simulink model "adcs_v16_integral_light_sun_sgp_igrf"  (Simulink 7.4)
settings: Solver=ode4  StartTime=0.0  StopTime=5000  FixedStep=s_SIM_STEP_SIZE  RelTol=1e-3
values from neighbouring files (symbols this model uses):
  A = ((T_SIDE + .29)*1e-3)^2    [constants_v13.m]    (also in constants_v15.m; constants_v15_Pow.m; constants_v15_Pow_ss_error.m; constants_v16_integral_kartavya.m)
  Bstar = SGP4dragp    (= -3.5889e-05)    [constants_v16_integral_light_sun_sgp_igrf_power_13Dec2011.m]    (also in getOrbitData.m = SGP4dragp; sgp.m = modTLE(4))
  Ca_Solar_Drag = 1.4    [constants_v13.m]    (also in constants_v15.m; constants_v15_Pow.m; constants_v15_Pow_ss_error.m; constants_v16_integral_kartavya.m)
  Cd = 2.2    [constants_v13.m]    (also in constants_v15.m; constants_v15_Pow.m; constants_v15_Pow_ss_error.m; constants_v16_integral_kartavya.m)
  check_time = 60000    [constants_v13.m]    (also in constants_v15.m = 10000; constants_v15_Pow.m = 10000; constants_v15_Pow_ss_error.m = 10000; constants_v16_integral_kartavya.m = 10000)
  ddn0 = 6*2*pi*SGPdragp2/(1440^3)    (= 0)    [constants_v16_integral_light_sun_sgp_igrf_power_13Dec2011.m]    (also in getOrbitData.m = 6*2*pi*SGPdragp2/(1440^3); sgp.m = modTLE(3))
  dn0 = 2*2*pi*SGPdragp1/(1440^2)    (= -4.7632944169e-11)    [constants_v16_integral_light_sun_sgp_igrf_power_13Dec2011.m]    (also in getOrbitData.m = 2*2*pi*SGPdragp1/(1440^2); sgp.m = modTLE(2))
  equinox = datenum('21-Mar-2010 12:0:0')    [constants_v13.m]    (also in constants_v15.m; constants_v15_Pow.m; constants_v15_Pow_ss_error.m; constants_v16_integral_kartavya.m)
  err_SGP = 0    [constants_v16_integral_kartavya.m]    (also in constants_v16_integral_light_sun_sgp_igrf_power_13Dec2011.m)
  i0 = pi*orbInc/180    (= 1.72229090587)    [constants_v16_integral_light_sun_sgp_igrf_power_13Dec2011.m]    (also in getOrbitData.m = pi*orbInc/180; sgp.m = modTLE(5))
  I_MAX = 0.5    [constants_v13.m]    (also in constants_v15.m; constants_v15_Pow.m; constants_v15_Pow_ss_error.m; constants_v16_integral_kartavya.m)
  I_TORQUER = 3.6 / 7.31    (= 0.492476060192)    [constants_v13.m]    (also in constants_v15.m; constants_v15_Pow.m; constants_v15_Pow_ss_error.m; constants_v16_integral_kartavya.m)
  Kd = 2* m_INERTIA / (s_numOrbits * T_ORBIT )    [constants_v13.m]    (also in constants_v15.m = m_INERTIA * (2 + delta)* zeta * w; constants_v15_Pow.m = m_INERTIA * (2 + delta)* zeta * w; constants_v15_Pow_ss_error.m = m_INERTIA * (2 + delta)* zeta * w; constants_v16_integral_kartavya.m = m_INERTIA * (2 + delta)* zeta * w)
  Kdetumb = K_det*eye(3)    [constants_v13.m]    (also in constants_v15.m; constants_v15_Pow.m; constants_v15_Pow_ss_error.m; constants_v16_integral_kartavya.m)
  Ki = m_INERTIA * delta * zeta * w^3    [constants_v15.m]    (also in constants_v15_Pow.m; constants_v15_Pow_ss_error.m; constants_v16_integral_kartavya.m; constants_v16_integral_light_sun_sgp_igrf_power_13Dec2011.m)
  Kp = m_INERTIA / (s_numOrbits * T_ORBIT * zeta)^2    [constants_v13.m]    (also in constants_v15.m = m_INERTIA * (w*w + 2*delta*zeta^2*w^2); constants_v15_Pow.m = m_INERTIA * (w*w + 2*delta*zeta^2*w^2); constants_v15_Pow_ss_error.m = m_INERTIA * (w*w + 2*delta*zeta^2*w^2); constants_v16_integral_kartavya.m = m_INERTIA * (w*w + 2*delta*zeta^2*w^2))
  M0 = pi*meanAno/180    (= 0)    [constants_v16_integral_light_sun_sgp_igrf_power_13Dec2011.m]    (also in getOrbitData.m = pi*meanAno/180; sgp.m = modTLE(9))
  m_INERTIA = [Ixx Ixy Ixz; Ixy Iyy Iyz; Ixz Iyz Izz]    [constants_v13.m]    (also in constants_v15.m; constants_v15_Pow.m = 1*[Ixx Ixy Ixz; Ixy Iyy Iyz; Ixz Iyz Izz]; constants_v15_Pow_ss_error.m = 1*[Ixx Ixy Ixz; Ixy Iyy Iyz; Ixz Iyz Izz]; constants_v16_integral_kartavya.m)
  mu = 6.673e-11*5.9742e24    (= 398658366000000)    [constants_v13.m]    (also in constants_v15.m; constants_v15_Pow.m; constants_v15_Pow_ss_error.m; constants_v16_integral_kartavya.m)
  N = 40    [constants_v13.m]    (also in constants_v15.m; constants_v15_Pow.m; constants_v15_Pow_ss_error.m; constants_v16_integral_kartavya.m)
  n0 = 2*pi*meanMo/1440    [constants_v16_integral_light_sun_sgp_igrf_power_13Dec2011.m]    (also in getOrbitData.m; sgp.m = modTLE(10))
  Ohm0 = pi*rghtAsc/180    (= 3.21433797681)    [constants_v16_integral_light_sun_sgp_igrf_power_13Dec2011.m]    (also in getOrbitData.m = pi*rghtAsc/180; sgp.m = modTLE(6))
  P_momentum_flux_from_the_sun = 4.4e-6    (= 4.4e-06)    [constants_v13.m]    (also in constants_v15.m; constants_v15_Pow.m; constants_v15_Pow_ss_error.m; constants_v16_integral_kartavya.m)
  q_BI0 = euler2qBI(roll0,pitch0,yaw0)    [constants_v13.m]    (also in constants_v15.m; constants_v15_Pow.m; constants_v15_Pow_ss_error.m; constants_v16_integral_kartavya.m)
  revNo = 1    [constants_v16_integral_kartavya.m]    (also in constants_v16_integral_light_sun_sgp_igrf_power_13Dec2011.m; precalcs.m; sgp.m = modTLE(11))
  s_AU = 159597870610    [constants_v16_integral_kartavya.m]    (also in constants_v16_integral_light_sun_sgp_igrf_power_13Dec2011.m; light_calc.m)
  s_FRAME_SIZE = 2    [constants_v13.m]    (also in constants_v15.m; constants_v15_Pow.m; constants_v15_Pow_ss_error.m; constants_v16_integral_kartavya.m)
  s_m_MAX = 0.95    [constants_v13.m]    (also in constants_v15.m; constants_v15_Pow.m; constants_v15_Pow_ss_error.m; constants_v16_integral_kartavya.m)
  s_MAG_B = 2.5e-5    (= 2.5e-05)    [constants_v13.m]    (also in constants_v15.m; constants_v15_Pow.m; constants_v15_Pow_ss_error.m; constants_v16_integral_kartavya.m)
  s_MAGMETER_WEIGHT = .9    (= 0.9)    [constants_v13.m]    (also in constants_v15.m; constants_v15_Pow.m; constants_v15_Pow_ss_error.m; constants_v16_integral_kartavya.m)
  s_Rearth = 6378164    [constants_v16_integral_kartavya.m]    (also in constants_v16_integral_light_sun_sgp_igrf_power_13Dec2011.m; light_calc.m)
  s_Rsun = 695500000    [constants_v16_integral_kartavya.m]    (also in constants_v16_integral_light_sun_sgp_igrf_power_13Dec2011.m; light_calc.m)
  s_SIM_STEP_SIZE = 0.1    [constants_v13.m]    (also in constants_v15.m; constants_v15_Pow.m; constants_v15_Pow_ss_error.m; constants_v16_integral_kartavya.m)
  s_SS_ADC_gain = 5    [constants_v13.m]    (also in constants_v15.m; constants_v15_Pow.m; constants_v15_Pow_ss_error.m; constants_v16_integral_kartavya.m)
  s_SS_ADC_res = 2^12 - 1    (= 4095)    [constants_v13.m]    (also in constants_v15.m; constants_v15_Pow.m; constants_v15_Pow_ss_error.m; constants_v16_integral_kartavya.m)
  s_SS_MAX_ANGLE = 85    [constants_v13.m]    (also in constants_v15.m; constants_v15_Pow.m; constants_v15_Pow_ss_error.m; constants_v16_integral_kartavya.m)
  s_TAU_W = 60    [constants_v13.m]    (also in constants_v15.m; constants_v15_Pow.m; constants_v15_Pow_ss_error.m; constants_v16_integral_kartavya.m)
  s_x_MAGMETER_BIAS = 50e-9    (= 5e-08)    [constants_v13.m]    (also in constants_v15.m; constants_v15_Pow.m; constants_v15_Pow_ss_error.m; constants_v16_integral_kartavya.m)
  s_YEAR = sime(1) + (sime(2)*30 - 30 + sime(3))/365    [constants_v16_integral_kartavya.m]    (also in constants_v16_integral_light_sun_sgp_igrf_power_13Dec2011.m; precalcs.m)
  side = 0.26    [constants_v13.m]    (also in constants_v15.m; constants_v15_Pow.m; constants_v15_Pow_ss_error.m; constants_v16_integral_kartavya.m)
  Snum = 6    [constants_v13.m]    (also in constants_v15.m; constants_v15_Pow.m; constants_v15_Pow_ss_error.m; constants_v16_integral_kartavya.m)
  t0 = (EpYear*meanYearDays + EpJD + EpTime)*1440    [constants_v16_integral_light_sun_sgp_igrf_power_13Dec2011.m]    (also in getOrbitData.m; sgp.m = modTLE(1))
  TLE_epoch = datenum('18-Oct-2010 10:30:0')    [constants_v16_integral_kartavya.m]    (also in constants_v16_integral_light_sun_sgp_igrf_power_13Dec2011.m; precalcs.m)
  today = datenum('18-Oct-2010 10:30:0')    [constants_v13.m]    (also in constants_v15.m; constants_v15_Pow.m; constants_v15_Pow_ss_error.m; constants_v16_integral_kartavya.m)
  tol_q4 = 0.7    [constants_v13.m]    (also in constants_v15.m = 0.85; constants_v15_Pow.m = 0.85; constants_v15_Pow_ss_error.m = 0.85; constants_v16_integral_kartavya.m = 0.85)
  tol_w = 4e-3    (= 0.004)    [constants_v13.m]    (also in constants_v15.m; constants_v15_Pow.m; constants_v15_Pow_ss_error.m; constants_v16_integral_kartavya.m)
  tolw_n2d = 10e-3    (= 0.01)    [constants_v15.m]    (also in constants_v15_Pow.m; constants_v15_Pow_ss_error.m; constants_v16_integral_kartavya.m; constants_v16_integral_light_sun_sgp_igrf_power_13Dec2011.m)
  Ts_display = 6    [constants_v13.m]    (also in constants_v15.m; constants_v15_Pow.m; constants_v15_Pow_ss_error.m; constants_v16_integral_kartavya.m)
  v_COM_to_COP_b = [.2; 1.75; .2]*1e-2    [constants_v13.m]    (also in constants_v15.m; constants_v15_Pow.m; constants_v15_Pow_ss_error.m; constants_v16_integral_kartavya.m)
  v_S1 = [1 0 0]    [constants_v13.m]    (also in constants_v15.m; constants_v15_Pow.m; constants_v15_Pow_ss_error.m; constants_v16_integral_kartavya.m)
  v_S2 = [-1 0 0]    [constants_v13.m]    (also in constants_v15.m; constants_v15_Pow.m; constants_v15_Pow_ss_error.m; constants_v16_integral_kartavya.m)
  v_S3 = [0 1 0]    [constants_v13.m]    (also in constants_v15.m; constants_v15_Pow.m; constants_v15_Pow_ss_error.m; constants_v16_integral_kartavya.m)
  v_S4 = [0 -1 0]    [constants_v13.m]    (also in constants_v15.m; constants_v15_Pow.m; constants_v15_Pow_ss_error.m; constants_v16_integral_kartavya.m)
  v_S5 = [0 0 1]    [constants_v13.m]    (also in constants_v15.m; constants_v15_Pow.m; constants_v15_Pow_ss_error.m; constants_v16_integral_kartavya.m)
  v_S6 = [0 0 -1]    [constants_v13.m]    (also in constants_v15.m; constants_v15_Pow.m; constants_v15_Pow_ss_error.m; constants_v16_integral_kartavya.m)
  v_x_MOUNTING_THETA_ZYX_BODY_TORQUER = [1; 1; 1]* pi/180    [constants_v13.m]    (also in constants_v15.m; constants_v15_Pow.m; constants_v15_Pow_ss_error.m; constants_v16_integral_kartavya.m)
  w0 = pi*argPer/180    (= 0)    [constants_v16_integral_light_sun_sgp_igrf_power_13Dec2011.m]    (also in getOrbitData.m = pi*argPer/180; sgp.m = modTLE(8))
  wx0 = 2*pi/180    (= 0.0349065850399)    [constants_v13.m]    (also in constants_v15.m = 0.00174532925199; constants_v15_Pow.m = 1.74532925199e-05; constants_v15_Pow_ss_error.m = 2.01533262693e-05; constants_v16_integral_kartavya.m = 0.0174532925199)
  wy0 = 1*pi/180    (= 0.0174532925199)    [constants_v13.m]    (also in constants_v15.m = 0.00174532925199; constants_v15_Pow.m = 1.74532925199e-05; constants_v15_Pow_ss_error.m = 2.01533262693e-05; constants_v16_integral_kartavya.m = 0)
  wz0 = -2*pi/180    (= -0.0349065850399)    [constants_v13.m]    (also in constants_v15.m = 0.00174532925199; constants_v15_Pow.m = 1.74532925199e-05; constants_v15_Pow_ss_error.m = 2.01533262693e-05; constants_v16_integral_kartavya.m = -0.00872664625997)
undefined symbols (not defined in the file or in its folder): agh, agh41, dgh, dgh41
libraries: commnoisgen2 x7, simulink x4, aerolibutil x2, dspmtrx3 x1
(part 1 of 2)
settings Model: Creator=Jaideep  LastModifiedBy=satellite  ExtModeTrigDuration=100
settings SolverCC: AutoInsertRateTranBlk=on
settings DataIOCC: ExternalInput=constants_v13  SaveFinalState=on  SaveOutput=off  SaveState=on  StateSaveName=tmp_raccel_xout
settings OptimizationCC: EfficientMapNaN2IntZero=off
settings HardwareCC: TargetEndianess=LittleEndian  TargetHWDeviceType=MATLAB Host  ProdEqTarget=off
settings RTWCC: SystemTargetFile=raccel.tlc  TemplateMakefile=raccel_default_tmf  RTWVerbose=off  ProcessScript=raccel_make_rtw_hook
settings CodeAppCC: GenerateComments=off  MaxIdLength=128  SimulinkBlockComments=off
settings RaccelTargetCC: TargetFunctionLibrary=ANSI_C  ERTMultiwordTypeDef=System defined  ERTMultiwordLength=256  IsPILTarget=off  ParMdlRefBuildCompliant=off  GeneratePreprocessorConditionals=Disable all  ERTFirstTimeCompliant=off  MultiInstanceERTCode=off  EnableShiftOperators=on  PortableWordSizes=off  RTWCAPISignals=off  RTWCAPIParams=off

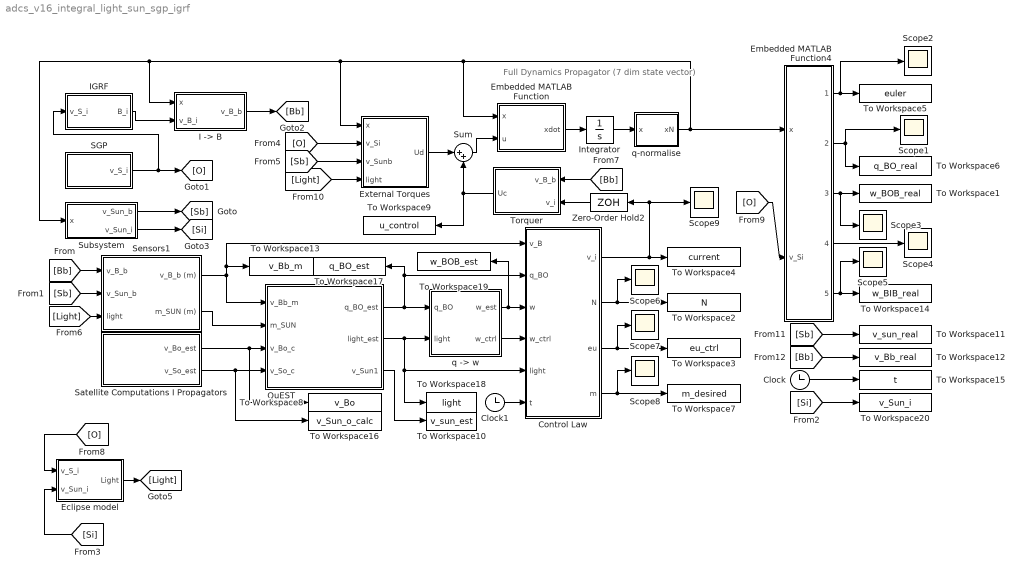
== system adcs_v16_integral_light_sun_sgp_igrf ==
  note: Full Dynamics Propagator
      |  (7 dim state vector)
  Clock : Clock
      settings: Decimation=10
  Clock1 : Clock
      settings: Decimation=10
  Control Law : Subsystem  TreatAsAtomicUnit=on  SystemSampleTime=s_FRAME_SIZE
  Eclipse model : Subsystem
  Embedded MATLAB Function : Stateflow chart
  Embedded MATLAB Function4 : Stateflow chart
  External Torques : Subsystem
  "I -> B" : Subsystem
  "IGRF " : Subsystem
  Integrator : Integrator  InitialCondition=[q_BI0; wx0; wy0; wz0]
  QuEST : Stateflow chart  TreatAsAtomicUnit=on  SystemSampleTime=s_FRAME_SIZE
  "SGP " : Subsystem
  Satellite Computations I Propagators : Subsystem  TreatAsAtomicUnit=on  SystemSampleTime=s_FRAME_SIZE
  Scope{1..9} (9 alike) : Scope
      Scope1 settings: YMin=-10  YMax=10  SaveName=ScopeData11  SampleInput=on  SampleTime=Ts_display
      Scope2 settings: YMin=-175  YMax=200  SaveName=ScopeData7  SampleInput=on  SampleTime=Ts_display
      Scope3 settings: YMin=-10  YMax=10  SaveName=ScopeData13  SampleInput=on  SampleTime=Ts_display
      Scope4 settings: YMin=-2.71051e-020  YMax=0.00035  SaveName=ScopeData14  SampleInput=on  SampleTime=Ts_display
      Scope5 settings: YMin=-10  YMax=10  SaveName=ScopeData15  SampleInput=on  SampleTime=Ts_display
      Scope6 settings: YMin=0  YMax=1  SaveName=ScopeData16  SampleInput=on  SampleTime=Ts_display
      Scope7 settings: YMin=-10  YMax=10  SaveName=ScopeData20  SampleInput=on  SampleTime=Ts_display
      Scope8 settings: YMin=-10  YMax=10  SaveName=ScopeData21  SampleInput=on  SampleTime=Ts_display
      Scope9 settings: YMin=-10  YMax=10  SaveName=ScopeData23  SampleInput=on  SampleTime=Ts_display
  Sensors1 : Subsystem
  Subsystem : Subsystem
  Sum : Sum  Inputs=|++  OutDataType=sfix(16)  OutScaling=2^0
  To Workspace1 : ToWorkspace  VariableName=w_BOB_real  SampleTime=Ts_display  SaveFormat=Array
  To Workspace10 : ToWorkspace  VariableName=v_sun_est  SampleTime=Ts_display  SaveFormat=Array
  To Workspace11 : ToWorkspace  VariableName=v_sun_real  SampleTime=Ts_display  SaveFormat=Array
  To Workspace12 : ToWorkspace  VariableName=v_Bb_real  SampleTime=Ts_display  SaveFormat=Array
  To Workspace13 : ToWorkspace  VariableName=v_Bb_m  SampleTime=Ts_display  SaveFormat=Array
  To Workspace14 : ToWorkspace  VariableName=w_BIB_real  SampleTime=Ts_display  SaveFormat=Array
  To Workspace15 : ToWorkspace  VariableName=t  SampleTime=Ts_display  SaveFormat=Array
  To Workspace16 : ToWorkspace  VariableName=v_Sun_o_calc  SampleTime=Ts_display  SaveFormat=Array
  To Workspace17 : ToWorkspace  VariableName=q_BO_est  SampleTime=Ts_display  SaveFormat=Array
  To Workspace18 : ToWorkspace  VariableName=light  SampleTime=Ts_display  SaveFormat=Array
  To Workspace19 : ToWorkspace  VariableName=w_BOB_est  SampleTime=Ts_display  SaveFormat=Array
  To Workspace2 : ToWorkspace  VariableName=N  SampleTime=Ts_display  SaveFormat=Array
  To Workspace20 : ToWorkspace  VariableName=v_Sun_i  SampleTime=Ts_display  SaveFormat=Array
  To Workspace3 : ToWorkspace  VariableName=eu_ctrl  SampleTime=Ts_display  SaveFormat=Array
  To Workspace4 : ToWorkspace  VariableName=current  SampleTime=Ts_display  SaveFormat=Array
  To Workspace5 : ToWorkspace  VariableName=euler  SampleTime=Ts_display  SaveFormat=Array
  To Workspace6 : ToWorkspace  VariableName=q_BO_real  SampleTime=Ts_display  SaveFormat=Array
  To Workspace7 : ToWorkspace  VariableName=m_desired  SampleTime=Ts_display  SaveFormat=Array
  To Workspace8 : ToWorkspace  VariableName=v_Bo  SampleTime=Ts_display  SaveFormat=Array
  To Workspace9 : ToWorkspace  VariableName=u_control  SampleTime=Ts_display  SaveFormat=Array
  Torquer : Subsystem
  Zero-Order Hold2 : ZeroOrderHold  SampleTime=s_FRAME_SIZE
  "q -> w" : Subsystem  TreatAsAtomicUnit=on  SystemSampleTime=s_FRAME_SIZE
  q-normalise : Stateflow chart
  wires:
  Embedded MATLAB Function/1(xdot) -> Integrator/1
  Integrator/1 -> q-normalise/1(x)
  "SGP "/1(v_S_i) -> [O], "IGRF "/1(v_S_i)
  q-normalise/1(xN) -> Subsystem/1(x), "I -> B"/1(x), External Torques/1(x), Embedded MATLAB Function/1(x), Embedded MATLAB Function4/1(x)
  Sum/1 -> Embedded MATLAB Function/2(u)
  "I -> B"/1(v_B_b) -> [Bb]
  Subsystem/1(v_Sun_b) -> [Sb]
  [Bb] -> Sensors1/1(v_B_b)
  [Sb] -> Sensors1/2(v_Sun_b)
  Subsystem/2(v_Sun_i) -> [Si]
  [O] -> External Torques/2(v_Si)
  [Sb] -> External Torques/3(v_Sunb)
  [Bb] -> Torquer/1(v_B_b)
  [Light] -> Sensors1/3(light)
  Sensors1/2(m_SUN (m)) -> QuEST/2(m_SUN)
  Sensors1/1(v_B_b (m)) -> QuEST/1(v_Bb_m), Control Law/1(v_B), To Workspace13/1
  Zero-Order Hold2/1 -> Torquer/2(v_i)
  Torquer/1(Uc) -> Sum/2, To Workspace9/1
  Satellite Computations I Propagators/1(v_Bo_est) -> To Workspace8/1, QuEST/3(v_Bo_c)
  Satellite Computations I Propagators/2(v_So_est) -> To Workspace16/1, QuEST/4(v_So_c)
  QuEST/1(q_BO_est) -> "q -> w"/1(q_BO), Control Law/2(q_BO), To Workspace17/1
  QuEST/2(light_est) -> "q -> w"/2(light), Control Law/5(light), To Workspace18/1
  Control Law/1(v_i) -> To Workspace4/1, Zero-Order Hold2/1, Scope9/1
  [O] -> Embedded MATLAB Function4/2(v_Si)
  Control Law/2(N) -> To Workspace2/1, Scope6/1
  Control Law/3(eu) -> To Workspace3/1, Scope7/1
  Control Law/4(m) -> To Workspace7/1, Scope8/1
  "q -> w"/1(w_est) -> Control Law/3(w), To Workspace19/1
  [Light] -> External Torques/4(light)
  "q -> w"/2(w_ctrl) -> Control Law/4(w_ctrl)
  QuEST/3(v_Sun1) -> To Workspace10/1
  [Sb] -> To Workspace11/1
  [Bb] -> To Workspace12/1
  Clock/1 -> To Workspace15/1
  Clock1/1 -> Control Law/6(t)
  Embedded MATLAB Function4/3(w_BOB) -> To Workspace1/1, Scope3/1
  Embedded MATLAB Function4/2(q_BO) -> To Workspace6/1, Scope1/1
  Embedded MATLAB Function4/1(euler) -> To Workspace5/1, Scope2/1
  Embedded MATLAB Function4/5(w_BIB) -> To Workspace14/1, Scope5/1
  Embedded MATLAB Function4/4(modw) -> Scope4/1
  [Si] -> To Workspace20/1
  External Torques/1(Ud) -> Sum/1
  [Si] -> Eclipse model/2(v_Sun_i)
  [O] -> Eclipse model/1(v_S_i)
  Eclipse model/1(Light) -> [Light]
  "IGRF "/1(B_i) -> "I -> B"/2(v_B_i)

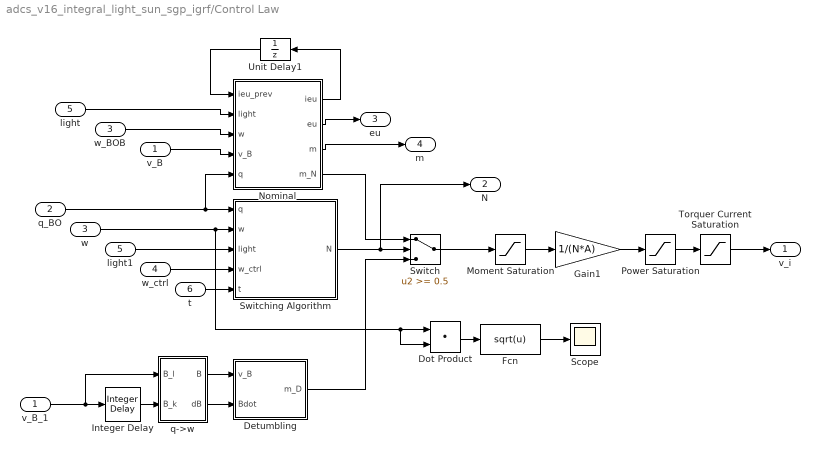
== system adcs_v16_integral_light_sun_sgp_igrf/Control Law ==
  v_B : Inport  OutDataType=sfix(16)  OutScaling=2^0
  q_BO : Inport  Port=2  OutDataType=sfix(16)  OutScaling=2^0
  w : Inport  Port=3  OutDataType=sfix(16)  OutScaling=2^0
  w_ctrl : Inport  Port=4  OutDataType=sfix(16)  OutScaling=2^0
  light : Inport  Port=5  OutDataType=sfix(16)  OutScaling=2^0
  t : Inport  Port=6  OutDataType=sfix(16)  OutScaling=2^0
  Detumbling : Stateflow chart
  Dot Product : DotProduct  OutDataType=fixdt(1, 16)  OutScaling=2^-10  InputSameDT=on  OutDataTypeStr=Inherit: Inherit via internal rule
  Fcn : Fcn  Expr=sqrt(u)
  Gain1 : Gain  Gain=1/(N*A)  ParameterDataType=sfix(16)  ParameterScaling=2^0  OutDataType=sfix(16)  OutScaling=2^0
  Integer Delay : simulink/Discrete/Integer Delay  vinit=0.0  samptime=-1  NumDelays=1
  Moment Saturation : Saturate  UpperLimit=s_m_MAX  LowerLimit=-s_m_MAX  OutDataType=sfix(16)  OutScaling=2^0
  Nominal : Stateflow chart
  Power Saturation : Saturate  UpperLimit=I_MAX  LowerLimit=-I_MAX  OutDataType=sfix(16)  OutScaling=2^0
  Scope : Scope
      settings: YMin=0  YMax=0.11  SaveName=ScopeData4
  Switch : Switch  Threshold=0.5  OutDataType=sfix(16)  OutScaling=2^0
  Switching Algorithm : Subsystem
  Torquer Current Saturation : Saturate  UpperLimit=I_TORQUER  LowerLimit=-I_TORQUER  OutDataType=sfix(16)  OutScaling=2^0
  Unit Delay1 : UnitDelay  X0=[0;0;0]  SampleTime=-1
  light1 : InportShadow  Port=5  OutDataType=sfix(16)  OutScaling=2^0  LatchByCopyingInsideSignal=off
  q->w : Stateflow chart
  v_B_1 : InportShadow  Port=1  OutDataType=sfix(16)  OutScaling=2^0  LatchByCopyingInsideSignal=off
  w_BOB : InportShadow  Port=3  OutDataType=sfix(16)  OutScaling=2^0  LatchByCopyingInsideSignal=off
  v_i : Outport  OutDataType=sfix(16)  OutScaling=2^0
  N : Outport  Port=2  OutDataType=sfix(16)  OutScaling=2^0
  eu : Outport  Port=3  OutDataType=sfix(16)  OutScaling=2^0
  m : Outport  Port=4  OutDataType=sfix(16)  OutScaling=2^0
  wires:
  w_ctrl/1 -> Switching Algorithm/4(w_ctrl)
  Nominal/3(m) -> m/1
  Nominal/2(eu) -> eu/1
  w_BOB/1 -> Nominal/3(w)
  light1/1 -> Switching Algorithm/3(light)
  v_B/1 -> Nominal/4(v_B)
  q->w/2(dB) -> Detumbling/2(Bdot)
  v_B_1/1 -> Integer Delay/1, q->w/1(B_l)
  w/1 -> Switching Algorithm/2(w), Dot Product/1, Dot Product/2
  Nominal/4(m_N) -> Switch/1
  Switching Algorithm/1(N) -> Switch/2, N/1
  Detumbling/1(m_D) -> Switch/3
  Switch/1 -> Moment Saturation/1
  Power Saturation/1 -> Torquer Current Saturation/1
  Moment Saturation/1 -> Gain1/1
  Torquer Current Saturation/1 -> v_i/1
  Gain1/1 -> Power Saturation/1
  light/1 -> Nominal/2(light)
  q_BO/1 -> Switching Algorithm/1(q), Nominal/5(q)
  Integer Delay/1 -> q->w/2(B_k)
  q->w/1(B) -> Detumbling/1(v_B)
  t/1 -> Switching Algorithm/5(t)
  Dot Product/1 -> Fcn/1
  Fcn/1 -> Scope/1
  Unit Delay1/1 -> Nominal/1(ieu_prev)
  Nominal/1(ieu) -> Unit Delay1/1

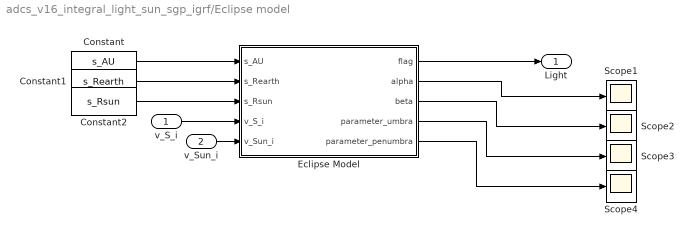
== system adcs_v16_integral_light_sun_sgp_igrf/Eclipse model ==
  v_S_i : Inport  OutDataType=sfix(16)  OutScaling=2^0
  v_Sun_i : Inport  Port=2  OutDataType=sfix(16)  OutScaling=2^0
  Constant : Constant  Value=s_AU  OutDataType=sfix(16)  OutScaling=2^0
  Constant1 : Constant  Value=s_Rearth  OutDataType=sfix(16)  OutScaling=2^0
  Constant2 : Constant  Value=s_Rsun  OutDataType=sfix(16)  OutScaling=2^0
  Eclipse Model : Stateflow chart
  Scope{1..4} (4 alike) : Scope
      Scope1 settings: TimeRange=80000  YMin=-6.5  YMax=1  SaveName=ScopeData3  SampleInput=on  SampleTime=5
      Scope2 settings: TimeRange=80000  YMin=-6.5  YMax=1  SaveName=ScopeData4  SampleInput=on  SampleTime=5
      Scope3 settings: TimeRange=80000  YMin=-6.5  YMax=1  SaveName=ScopeData5  SampleInput=on  SampleTime=5
      Scope4 settings: TimeRange=80000  YMin=-6.5  YMax=1  SaveName=ScopeData6  SampleInput=on  SampleTime=5
  Light : Outport  OutDataType=sfix(16)  OutScaling=2^0
  wires:
  Constant/1 -> Eclipse Model/1(s_AU)
  Constant1/1 -> Eclipse Model/2(s_Rearth)
  Constant2/1 -> Eclipse Model/3(s_Rsun)
  Eclipse Model/1(flag) -> Light/1
  v_S_i/1 -> Eclipse Model/4(v_S_i)
  v_Sun_i/1 -> Eclipse Model/5(v_Sun_i)
  Eclipse Model/2(alpha) -> Scope1/1
  Eclipse Model/3(beta) -> Scope2/1
  Eclipse Model/4(parameter_umbra) -> Scope3/1
  Eclipse Model/5(parameter_penumbra) -> Scope4/1

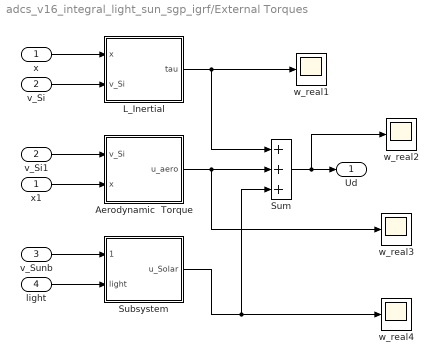
== system adcs_v16_integral_light_sun_sgp_igrf/External Torques ==
  x : Inport  OutDataType=sfix(16)  OutScaling=2^0
  v_Si : Inport  Port=2  OutDataType=sfix(16)  OutScaling=2^0
  v_Sunb : Inport  Port=3  OutDataType=sfix(16)  OutScaling=2^0
  light : Inport  Port=4  OutDataType=sfix(16)  OutScaling=2^0
  Aerodynamic  Torque : Subsystem
  L_Inertial : Stateflow chart
  Subsystem : Subsystem
  Sum : Sum  Inputs=+++  OutDataType=fixdt(1, 16)  OutScaling=2^0
  v_Si1 : InportShadow  Port=2  OutDataType=sfix(16)  OutScaling=2^0  LatchByCopyingInsideSignal=off
  w_real{1..4} (4 alike) : Scope
      w_real1 settings: TimeRange=80000  YMin=-3e-009  YMax=1.1e-008  SaveName=ScopeData18  SampleInput=on  SampleTime=5
      w_real2 settings: TimeRange=80000  YMin=-7e-009  YMax=1e-008  SaveName=ScopeData17  SampleInput=on  SampleTime=5
      w_real3 settings: YMin=-8e-010  YMax=1.4e-009  SaveName=ScopeData19  SampleInput=on  SampleTime=5
      w_real4 settings: YMin=-6e-009  YMax=1e-008  SaveName=ScopeData22  SampleInput=on  SampleTime=5
  x1 : InportShadow  Port=1  OutDataType=sfix(16)  OutScaling=2^0  LatchByCopyingInsideSignal=off
  Ud : Outport  OutDataType=sfix(16)  OutScaling=2^0
  wires:
  x/1 -> L_Inertial/1(x)
  v_Si/1 -> L_Inertial/2(v_Si)
  L_Inertial/1(tau) -> Sum/1, w_real1/1
  Aerodynamic  Torque/1(u_aero) -> Sum/2, w_real3/1
  x1/1 -> Aerodynamic  Torque/2(x)
  v_Si1/1 -> Aerodynamic  Torque/1(v_Si)
  Sum/1 -> Ud/1, w_real2/1
  v_Sunb/1 -> Subsystem/1(v_Sun_b)
  Subsystem/1(u_Solar) -> Sum/3, w_real4/1
  light/1 -> Subsystem/2(light)

== system adcs_v16_integral_light_sun_sgp_igrf/I -> B ==
  x : Inport  OutDataType=sfix(16)  OutScaling=2^0
  v_B_i : Inport  Port=2  OutDataType=sfix(16)  OutScaling=2^0
  Gain : Gain  Gain=1e-9  ParameterDataType=fixdt(1, 16)  ParameterScaling=2^0  OutDataType=fixdt(1, 16)  OutScaling=2^0
  L_Inertial : Stateflow chart
  v_B_b : Outport  OutDataType=sfix(16)  OutScaling=2^0
  wires:
  L_Inertial/1(v_B) -> v_B_b/1
  x/1 -> L_Inertial/1(x)
  v_B_i/1 -> Gain/1
  Gain/1 -> L_Inertial/2(v_I)

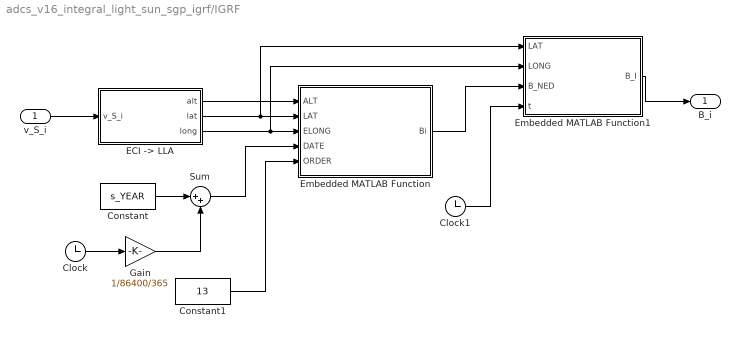
== system adcs_v16_integral_light_sun_sgp_igrf/IGRF  ==
  v_S_i : Inport  OutDataType=fixdt(1, 16)  OutScaling=2^0
  Clock : Clock
      settings: Decimation=10
  Clock1 : Clock
      settings: Decimation=10
  Constant : Constant  Value=s_YEAR  OutDataType=fixdt(1, 16)  OutScaling=2^0
  Constant1 : Constant  Value=13  OutDataType=fixdt(1, 16)  OutScaling=2^0
  "ECI -> LLA" : Subsystem
  Embedded MATLAB Function : Stateflow chart
  Embedded MATLAB Function1 : Stateflow chart
  Gain : Gain  Gain=1/86400/365  ParameterDataType=fixdt(1, 16)  ParameterScaling=2^0  OutDataType=fixdt(1, 16)  OutScaling=2^0
  Sum : Sum  Inputs=|++  OutDataType=fixdt(1, 16)  OutScaling=2^0
  B_i : Outport  OutDataType=fixdt(1, 16)  OutScaling=2^0
  wires:
  v_S_i/1 -> "ECI -> LLA"/1(v_S_i)
  "ECI -> LLA"/1(alt) -> Embedded MATLAB Function/1(ALT)
  "ECI -> LLA"/2(lat) -> Embedded MATLAB Function/2(LAT), Embedded MATLAB Function1/1(LAT)
  "ECI -> LLA"/3(long) -> Embedded MATLAB Function/3(ELONG), Embedded MATLAB Function1/2(LONG)
  Clock/1 -> Gain/1
  Constant/1 -> Sum/1
  Gain/1 -> Sum/2
  Sum/1 -> Embedded MATLAB Function/4(DATE)
  Constant1/1 -> Embedded MATLAB Function/5(ORDER)
  Embedded MATLAB Function/1(Bi) -> Embedded MATLAB Function1/3(B_NED)
  Embedded MATLAB Function1/1(B_I) -> B_i/1
  Clock1/1 -> Embedded MATLAB Function1/4(t)

== system adcs_v16_integral_light_sun_sgp_igrf/SGP  ==
  note: SGP
  Add : Sum  OutDataType=sfix(16)  OutScaling=2^-10
  Add1 : Sum  OutDataType=sfix(16)  OutScaling=2^-10
  Clock : Clock
      settings: Decimation=10
  Constant : Constant  Value=err_SGP  VectorParams1D=off  OutDataType=sfix(16)  OutScaling=2^0
  Constant1 : Constant  Value=(today - TLE_epoch) * 86400  VectorParams1D=off  OutDataType=sfix(16)  OutScaling=2^0
  Gain : Gain  Gain=1/60  ParameterDataType=sfix(16)  ParameterScaling=2^0  OutDataType=sfix(16)  OutScaling=2^0
  Gain1 : Gain  Gain=0  ParameterDataType=sfix(16)  ParameterScaling=2^0  OutDataType=sfix(16)  OutScaling=2^0
  Mux : Mux  Inputs=2
  Subsystem : Subsystem
  Transpose : dspmtrx3/Transpose  SystemSampleTime=-1  Hermitian=off  overflowFlag=off
  v_S_i : Outport  OutDataType=sfix(16)  OutScaling=2^0
  wires:
  Transpose/1 -> v_S_i/1
  Gain1/1 -> Add/1
  Add1/1 -> Gain/1
  Clock/1 -> Add1/2
  Constant1/1 -> Add1/1
  Add/1 -> Transpose/1
  Constant/1 -> Gain1/1
  Gain/1 -> Subsystem/1(dt)
  Mux/1 -> Add/2
  Subsystem/2(V (m/s)) -> Mux/2
  Subsystem/1(R (m)) -> Mux/1

== system adcs_v16_integral_light_sun_sgp_igrf/Satellite Computations I Propagators ==
  From File : FromFile  FileName=Si_120k
  From File2 : FromFile  FileName=SGP_est_120k
  From File3 : FromFile  FileName=Bi8_est_120k
  m_TOI_NEW : Stateflow chart
  m_TOI_NEW1 : Stateflow chart
  v_Bo_est : Outport  OutDataType=sfix(16)  OutScaling=2^0
  v_So_est : Outport  Port=2  OutDataType=sfix(16)  OutScaling=2^0
  wires:
  From File3/1 -> m_TOI_NEW/2(v_I)
  From File2/1 -> m_TOI_NEW1/2(ECI), m_TOI_NEW/1(ECI)
  From File/1 -> m_TOI_NEW1/1(v_I)
  m_TOI_NEW/1(v_O) -> v_Bo_est/1
  m_TOI_NEW1/1(v_O) -> v_So_est/1

== system adcs_v16_integral_light_sun_sgp_igrf/Sensors1 ==
  note: 'm' stands for measured
  v_B_b : Inport  OutDataType=sfix(16)  OutScaling=2^0
  v_Sun_b : Inport  Port=2  OutDataType=sfix(16)  OutScaling=2^0
  light : Inport  Port=3  OutDataType=sfix(16)  OutScaling=2^0
  Magnetometer simple : Subsystem
  Sun Sensors : Subsystem
  v_B_b (m) : Outport  OutDataType=sfix(16)  OutScaling=2^0
  m_SUN (m) : Outport  Port=2  OutDataType=sfix(16)  OutScaling=2^0
  wires:
  light/1 -> Sun Sensors/2(Light)
  Magnetometer simple/1(v_B_b(m)) -> v_B_b (m)/1
  v_B_b/1 -> Magnetometer simple/1(v_B_b)
  v_Sun_b/1 -> Sun Sensors/1(v_Sun_b)
  Sun Sensors/1(m_SUN) -> m_SUN (m)/1

== system adcs_v16_integral_light_sun_sgp_igrf/Subsystem ==
  x : Inport  OutDataType=sfix(16)  OutScaling=2^0
  Clock : Clock
      settings: Decimation=10
  Constant : Constant  Value=today  OutDataType=sfix(16)  OutScaling=2^0
  Constant1 : Constant  Value=equinox  OutDataType=sfix(16)  OutScaling=2^0
  Sun Vector Propagator : Stateflow chart
  f: I->B : Stateflow chart
  v_Sun_b : Outport  OutDataType=sfix(16)  OutScaling=2^0
  v_Sun_i : Outport  Port=2  OutDataType=sfix(16)  OutScaling=2^0
  wires:
  x/1 -> f: I->B/1(x)
  f: I->B/1(v_B) -> v_Sun_b/1
  Sun Vector Propagator/1(v_Sun_i) -> f: I->B/2(v_I), v_Sun_i/1
  Clock/1 -> Sun Vector Propagator/2(t)
  Constant/1 -> Sun Vector Propagator/1(today)
  Constant1/1 -> Sun Vector Propagator/3(equinox)

== system adcs_v16_integral_light_sun_sgp_igrf/Torquer ==
  v_B_b : Inport  OutDataType=sfix(16)  OutScaling=2^0
  v_i : Inport  Port=2  OutDataType=sfix(16)  OutScaling=2^0
  3x3 Cross Product : aerolibutil/3x3 Cross Product  SystemSampleTime=-1
  Constant : Constant  Value=v_x_MOUNTING_THETA_ZYX_BODY_TORQUER  OutDataType=sfix(16)  OutScaling=2^0
  Embedded MATLAB Function4 : Stateflow chart
  Gain : Gain  Gain=0  ParameterDataType=sfix(16)  ParameterScaling=2^0  OutDataType=sfix(16)  OutScaling=2^0
  Gain2 : Gain  Gain=N*A  ParameterDataType=sfix(16)  ParameterScaling=2^0  OutDataType=sfix(16)  OutScaling=2^0
  PWM : Quantizer  QuantizationInterval=s_PWM_RES
  Product : Product  Multiplication=Matrix(*)  OutDataType=sfix(16)  OutScaling=2^0  RndMeth=Zero
  Uc : Outport  OutDataType=sfix(16)  OutScaling=2^0
  wires:
  PWM/1 -> Gain2/1
  v_B_b/1 -> 3x3 Cross Product/2
  3x3 Cross Product/1 -> Uc/1
  v_i/1 -> PWM/1
  Embedded MATLAB Function4/1(DCM) -> Product/1
  Gain2/1 -> Product/2
  Product/1 -> 3x3 Cross Product/1
  Constant/1 -> Gain/1
  Gain/1 -> Embedded MATLAB Function4/1(euler)

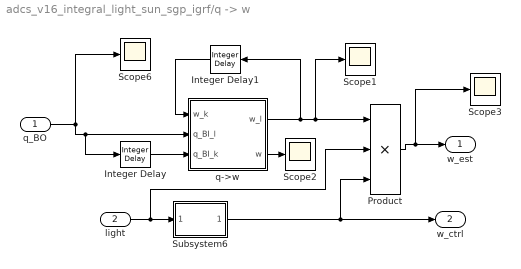
== system adcs_v16_integral_light_sun_sgp_igrf/q -> w ==
  q_BO : Inport
  light : Inport  Port=2
  Integer Delay : simulink/Discrete/Integer Delay  vinit=0.0  samptime=-1  NumDelays=1
  Integer Delay1 : simulink/Discrete/Integer Delay  vinit=[0;0;0]  samptime=-1  NumDelays=1
  Product : Product  Inputs=3  OutDataType=fixdt(1, 16)  OutScaling=2^0  RndMeth=Zero
  Scope{1..3,6} (4 alike) : Scope
      Scope1 settings: YMin=-10  YMax=10  SaveName=ScopeData9  SampleInput=on
      Scope2 settings: YMin=-10  YMax=10  SaveName=ScopeData10  SampleInput=on
      Scope3 settings: YMin=-10  YMax=10  SaveName=ScopeData12  SampleInput=on
      Scope6 settings: YMin=-10  YMax=10  SaveName=ScopeData8  SampleInput=on
  Subsystem6 : Subsystem
  q->w : Stateflow chart
  w_est : Outport
  w_ctrl : Outport  Port=2
  wires:
  Subsystem6/1(w-ctrl) -> w_ctrl/1, Product/3
  q_BO/1 -> Integer Delay/1, q->w/2(q_BI_l), Scope6/1
  light/1 -> Product/2, Subsystem6/1(light)
  Product/1 -> w_est/1, Scope3/1
  Integer Delay/1 -> q->w/3(q_BI_k)
  q->w/1(w_l) -> Integer Delay1/1, Product/1, Scope1/1
  Integer Delay1/1 -> q->w/1(w_k)
  q->w/2(w) -> Scope2/1

== system adcs_v16_integral_light_sun_sgp_igrf/Control Law/Switching Algorithm ==
  note: remov the t=0 checking
      | code, not necessary
  q : Inport  OutDataType=sfix(16)  OutScaling=2^0
  w : Inport  Port=2  OutDataType=sfix(16)  OutScaling=2^0
  light : Inport  Port=3  OutDataType=sfix(16)  OutScaling=2^0
  w_ctrl : Inport  Port=4  OutDataType=sfix(16)  OutScaling=2^0
  t : Inport  Port=5  OutDataType=sfix(16)  OutScaling=2^0
  Scope1 : Scope
      settings: TimeRange=140000  YMin=0  YMax=1.3  SaveName=ScopeData5
  Unit Delay : UnitDelay  SampleTime=-1
  Unit Delay1 : UnitDelay  SampleTime=-1
  gate pulse : Stateflow chart
  N : Outport  OutDataType=sfix(16)  OutScaling=2^0
  wires:
  t/1 -> gate pulse/4(t)
  w_ctrl/1 -> gate pulse/6(w_ctrl)
  light/1 -> gate pulse/5(light_flag)
  gate pulse/1(N) -> N/1, Unit Delay1/1
  q/1 -> gate pulse/3(q)
  gate pulse/3(t_now) -> Unit Delay/1
  w/1 -> gate pulse/2(w)
  Unit Delay/1 -> gate pulse/7(t_now_prev)
  Unit Delay1/1 -> gate pulse/1(N_prev)
  gate pulse/2(P) -> Scope1/1

== system adcs_v16_integral_light_sun_sgp_igrf/External Torques/Aerodynamic  Torque ==
  v_Si : Inport
  x : Inport  Port=2
  Demux : Demux  Outputs=2
  aero torque : Stateflow chart
  v_I to v_B : Stateflow chart
  u_aero : Outport  OutDataType=sfix(16)  OutScaling=2^0
  wires:
  v_I to v_B/1(v_B) -> aero torque/2(v_B)
  v_Si/1 -> Demux/1
  Demux/2 -> v_I to v_B/1(v_I)
  x/1 -> v_I to v_B/2(x)
  aero torque/1(u_aero) -> u_aero/1

== system adcs_v16_integral_light_sun_sgp_igrf/External Torques/Subsystem ==
  v_Sun_b : Inport  OutDataType=sfix(16)  OutScaling=2^0
  light : Inport  Port=2  OutDataType=sfix(16)  OutScaling=2^0
  Solar_drag : Stateflow chart
  Vector from CoM to CoP_in Body frame (yet to be finalized)2 : Constant  Value=v_COM_to_COP_b  VectorParams1D=off  OutDataType=sfix(16)  OutScaling=2^0
  _ : aerolibutil/3x3 Cross Product  SystemSampleTime=-1
  u_Solar : Outport  OutDataType=sfix(16)  OutScaling=2^0
  wires:
  _/1 -> u_Solar/1
  v_Sun_b/1 -> Solar_drag/1(v_Sun_b)
  light/1 -> Solar_drag/2(light)
  Solar_drag/1(solar_drag) -> _/2
  Vector from CoM to CoP_in Body frame (yet to be finalized)2/1 -> _/1

== system adcs_v16_integral_light_sun_sgp_igrf/IGRF /ECI -> LLA ==
  v_S_i : Inport
  Clock2 : Clock
      settings: Decimation=10
  "r_ECEF -> r_LLA" : Stateflow chart
  "r_ECI -> r_ECEF" : Stateflow chart
  alt : Outport
  lat : Outport  Port=2
  long : Outport  Port=3
  wires:
  "r_ECEF -> r_LLA"/3(Altitude) -> alt/1
  "r_ECEF -> r_LLA"/2(Longitude) -> long/1
  v_S_i/1 -> "r_ECI -> r_ECEF"/1(v_S_i)
  "r_ECEF -> r_LLA"/1(Latitude) -> lat/1
  "r_ECI -> r_ECEF"/1(r_ECEF) -> "r_ECEF -> r_LLA"/1(r_ECEF)
  Clock2/1 -> "r_ECI -> r_ECEF"/2(t)

== system adcs_v16_integral_light_sun_sgp_igrf/SGP /Subsystem ==
  dt : Inport
  Embedded MATLAB Function2 : Stateflow chart
  R (m) : Outport
  V (m/s) : Outport  Port=2
  wires:
  Embedded MATLAB Function2/2(dR) -> V (m/s)/1
  dt/1 -> Embedded MATLAB Function2/1(dT)
  Embedded MATLAB Function2/1(R) -> R (m)/1

== system adcs_v16_integral_light_sun_sgp_igrf/Sensors1/Magnetometer simple ==
  v_B_b : Inport  OutDataType=sfix(16)  OutScaling=2^0
  Constant : Constant  Value=s_x_MAGMETER_BIAS  OutDataType=fixdt(1, 16)  OutScaling=2^0
  Gaussian Noise Generator : commnoisgen2/Gaussian Noise Generator  SystemSampleTime=-1  m=0  d=s_x_MAGMETER  s=41  Ts=s_SIM_STEP_SIZE  frameBased=off  sampPerFrame=1  orient=off  outDataType=double
  Sum1 : Sum  Inputs=+++  OutDataType=sfix(16)  OutScaling=2^0
  v_B_b(m) : Outport  OutDataType=sfix(16)  OutScaling=2^0
  wires:
  Constant/1 -> Sum1/3
  Sum1/1 -> v_B_b(m)/1
  Gaussian Noise Generator/1 -> Sum1/1
  v_B_b/1 -> Sum1/2

== system adcs_v16_integral_light_sun_sgp_igrf/Sensors1/Sun Sensors ==
  v_Sun_b : Inport  OutDataType=sfix(16)  OutScaling=2^0
  Light : Inport  Port=2  OutDataType=sfix(16)  OutScaling=2^0
  Embedded MATLAB Function : Stateflow chart
  S1 : Subsystem
  S2 : Subsystem
  S3 : Subsystem
  S4 : Subsystem
  S5 : Subsystem
  S6 : Subsystem
  m_SUN : Outport  OutDataType=fixdt(1, 16)  OutScaling=2^0
  wires:
  Embedded MATLAB Function/1(m_SUN) -> m_SUN/1
  v_Sun_b/1 -> S6/2(v_Sunb), S5/2(v_Sunb), S4/2(v_Sunb), S3/2(v_Sunb), S2/2(v_Sunb), S1/2(v_Sunb)
  S1/1(v_S) -> Embedded MATLAB Function/1(v_S1)
  S1/2(s_S) -> Embedded MATLAB Function/2(s_S1)
  S2/1(v_S) -> Embedded MATLAB Function/3(v_S2)
  S2/2(s_S) -> Embedded MATLAB Function/4(s_S2)
  S3/1(v_S) -> Embedded MATLAB Function/5(v_S3)
  S3/2(s_S) -> Embedded MATLAB Function/6(s_S3)
  S4/1(v_S) -> Embedded MATLAB Function/7(v_S4)
  S4/2(s_S) -> Embedded MATLAB Function/8(s_S4)
  S5/1(v_S) -> Embedded MATLAB Function/9(v_S5)
  S5/2(s_S) -> Embedded MATLAB Function/10(s_S5)
  S6/1(v_S) -> Embedded MATLAB Function/11(v_S6)
  S6/2(s_S) -> Embedded MATLAB Function/12(s_S6)
  Light/1 -> S1/1(light), S2/1(light), S3/1(light), S4/1(light), S5/1(light), S6/1(light)

== system adcs_v16_integral_light_sun_sgp_igrf/q -> w/Subsystem6 ==
  light : Inport  OutDataType=fixdt(1, 16)  OutScaling=2^0
  (1-L) + L/z : Stateflow chart
  Integer Delay : simulink/Discrete/Integer Delay  vinit=0.0  samptime=-1  NumDelays=300
  Scope : Scope
  Scope1 : Scope
  Scope2 : Scope
      settings: TimeRange=80000  SaveName=ScopeData2
  w-ctrl : Outport  OutDataType=fixdt(1, 16)  OutScaling=2^0
  wires:
  (1-L) + L/z/1(y) -> Scope/1, w-ctrl/1
  light/1 -> (1-L) + L/z/1(a), Integer Delay/1, Scope2/1
  Integer Delay/1 -> Scope1/1, (1-L) + L/z/2(b)

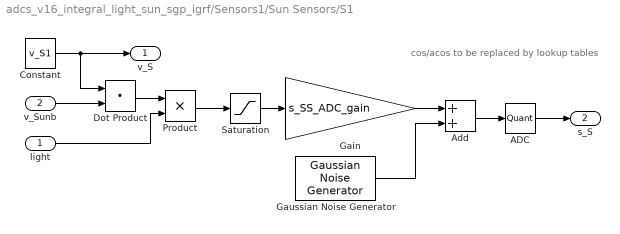
== system adcs_v16_integral_light_sun_sgp_igrf/Sensors1/Sun Sensors/S1 ==
  note: cos/acos to be replaced by lookup tables
  light : Inport  OutDataType=sfix(16)  OutScaling=2^0
  v_Sunb : Inport  Port=2  OutDataType=sfix(16)  OutScaling=2^0
  ADC : Quantizer  QuantizationInterval=1/s_SS_ADC_res
  Add : Sum  OutDataType=sfix(16)  OutScaling=2^-10
  Constant : Constant  Value=v_S1  OutDataType=sfix(16)  OutScaling=2^0
  Dot Product : DotProduct  OutDataType=sfix(16)  OutScaling=2^-10  InputSameDT=on  OutDataTypeStr=Inherit: Inherit via internal rule
  Gain : Gain  Gain=s_SS_ADC_gain  ParameterDataType=sfix(16)  ParameterScaling=2^0  OutDataType=sfix(16)  OutScaling=2^0
  Gaussian Noise Generator : commnoisgen2/Gaussian Noise Generator  SystemSampleTime=-1  m=0  d=s_x_SUNSENSOR  s=41  Ts=s_SIM_STEP_SIZE  frameBased=off  sampPerFrame=1  orient=off  outDataType=double
  Product : Product  OutDataType=fixdt(1, 16)  OutScaling=2^0  RndMeth=Zero
  Saturation : Saturate  UpperLimit=inf  LowerLimit=0  OutDataType=sfix(16)  OutScaling=2^0
  v_S : Outport  OutDataType=sfix(16)  OutScaling=2^0
  s_S : Outport  Port=2  OutDataType=sfix(16)  OutScaling=2^0
  wires:
  light/1 -> Product/2
  Product/1 -> Saturation/1
  Dot Product/1 -> Product/1
  v_Sunb/1 -> Dot Product/2
  Saturation/1 -> Gain/1
  Constant/1 -> v_S/1, Dot Product/1
  Gaussian Noise Generator/1 -> Add/2
  Gain/1 -> Add/1
  Add/1 -> ADC/1
  ADC/1 -> s_S/1

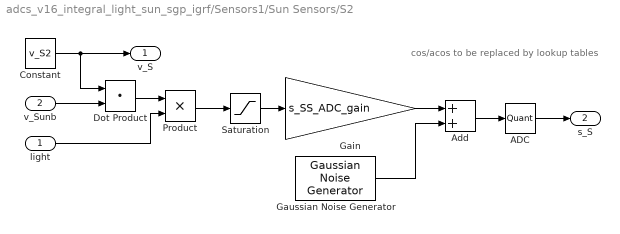
== system adcs_v16_integral_light_sun_sgp_igrf/Sensors1/Sun Sensors/S2 ==
  note: cos/acos to be replaced by lookup tables
  light : Inport  OutDataType=sfix(16)  OutScaling=2^0
  v_Sunb : Inport  Port=2  OutDataType=sfix(16)  OutScaling=2^0
  ADC : Quantizer  QuantizationInterval=1/s_SS_ADC_res
  Add : Sum  OutDataType=sfix(16)  OutScaling=2^-10
  Constant : Constant  Value=v_S2  OutDataType=sfix(16)  OutScaling=2^0
  Dot Product : DotProduct  OutDataType=sfix(16)  OutScaling=2^-10  InputSameDT=on  OutDataTypeStr=Inherit: Inherit via internal rule
  Gain : Gain  Gain=s_SS_ADC_gain  ParameterDataType=sfix(16)  ParameterScaling=2^0  OutDataType=sfix(16)  OutScaling=2^0
  Gaussian Noise Generator : commnoisgen2/Gaussian Noise Generator  SystemSampleTime=-1  m=0  d=s_x_SUNSENSOR  s=41  Ts=s_SIM_STEP_SIZE  frameBased=off  sampPerFrame=1  orient=off  outDataType=double
  Product : Product  OutDataType=fixdt(1, 16)  OutScaling=2^0  RndMeth=Zero
  Saturation : Saturate  UpperLimit=inf  LowerLimit=0  OutDataType=sfix(16)  OutScaling=2^0
  v_S : Outport  OutDataType=sfix(16)  OutScaling=2^0
  s_S : Outport  Port=2  OutDataType=sfix(16)  OutScaling=2^0
  wires:
  ADC/1 -> s_S/1
  Add/1 -> ADC/1
  Gain/1 -> Add/1
  Gaussian Noise Generator/1 -> Add/2
  Constant/1 -> Dot Product/1, v_S/1
  Saturation/1 -> Gain/1
  v_Sunb/1 -> Dot Product/2
  Dot Product/1 -> Product/1
  Product/1 -> Saturation/1
  light/1 -> Product/2

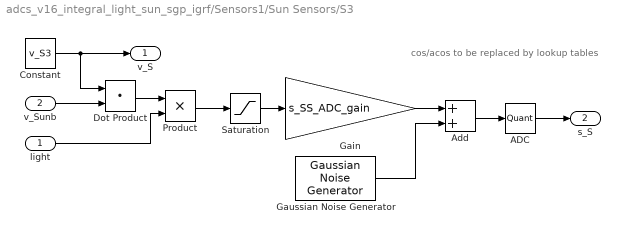
== system adcs_v16_integral_light_sun_sgp_igrf/Sensors1/Sun Sensors/S3 ==
  note: cos/acos to be replaced by lookup tables
  light : Inport  OutDataType=sfix(16)  OutScaling=2^0
  v_Sunb : Inport  Port=2  OutDataType=sfix(16)  OutScaling=2^0
  ADC : Quantizer  QuantizationInterval=1/s_SS_ADC_res
  Add : Sum  OutDataType=sfix(16)  OutScaling=2^-10
  Constant : Constant  Value=v_S3  OutDataType=sfix(16)  OutScaling=2^0
  Dot Product : DotProduct  OutDataType=sfix(16)  OutScaling=2^-10  InputSameDT=on  OutDataTypeStr=Inherit: Inherit via internal rule
  Gain : Gain  Gain=s_SS_ADC_gain  ParameterDataType=sfix(16)  ParameterScaling=2^0  OutDataType=sfix(16)  OutScaling=2^0
  Gaussian Noise Generator : commnoisgen2/Gaussian Noise Generator  SystemSampleTime=-1  m=0  d=s_x_SUNSENSOR  s=41  Ts=s_SIM_STEP_SIZE  frameBased=off  sampPerFrame=1  orient=off  outDataType=double
  Product : Product  OutDataType=fixdt(1, 16)  OutScaling=2^0  RndMeth=Zero
  Saturation : Saturate  UpperLimit=inf  LowerLimit=0  OutDataType=sfix(16)  OutScaling=2^0
  v_S : Outport  OutDataType=sfix(16)  OutScaling=2^0
  s_S : Outport  Port=2  OutDataType=sfix(16)  OutScaling=2^0
  wires:
  light/1 -> Product/2
  Product/1 -> Saturation/1
  Dot Product/1 -> Product/1
  v_Sunb/1 -> Dot Product/2
  Saturation/1 -> Gain/1
  Constant/1 -> v_S/1, Dot Product/1
  Gaussian Noise Generator/1 -> Add/2
  Gain/1 -> Add/1
  Add/1 -> ADC/1
  ADC/1 -> s_S/1

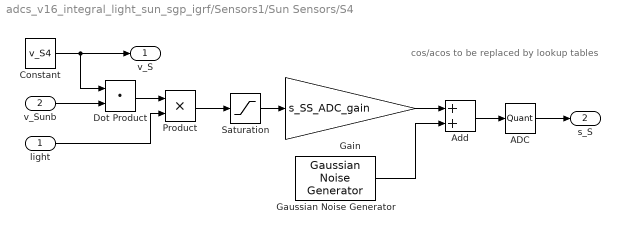
== system adcs_v16_integral_light_sun_sgp_igrf/Sensors1/Sun Sensors/S4 ==
  note: cos/acos to be replaced by lookup tables
  light : Inport  OutDataType=sfix(16)  OutScaling=2^0
  v_Sunb : Inport  Port=2  OutDataType=sfix(16)  OutScaling=2^0
  ADC : Quantizer  QuantizationInterval=1/s_SS_ADC_res
  Add : Sum  OutDataType=sfix(16)  OutScaling=2^-10
  Constant : Constant  Value=v_S4  OutDataType=sfix(16)  OutScaling=2^0
  Dot Product : DotProduct  OutDataType=sfix(16)  OutScaling=2^-10  InputSameDT=on  OutDataTypeStr=Inherit: Inherit via internal rule
  Gain : Gain  Gain=s_SS_ADC_gain  ParameterDataType=sfix(16)  ParameterScaling=2^0  OutDataType=sfix(16)  OutScaling=2^0
  Gaussian Noise Generator : commnoisgen2/Gaussian Noise Generator  SystemSampleTime=-1  m=0  d=s_x_SUNSENSOR  s=41  Ts=s_SIM_STEP_SIZE  frameBased=off  sampPerFrame=1  orient=off  outDataType=double
  Product : Product  OutDataType=fixdt(1, 16)  OutScaling=2^0  RndMeth=Zero
  Saturation : Saturate  UpperLimit=inf  LowerLimit=0  OutDataType=sfix(16)  OutScaling=2^0
  v_S : Outport  OutDataType=sfix(16)  OutScaling=2^0
  s_S : Outport  Port=2  OutDataType=sfix(16)  OutScaling=2^0
  wires:
  ADC/1 -> s_S/1
  Add/1 -> ADC/1
  Gain/1 -> Add/1
  Gaussian Noise Generator/1 -> Add/2
  Constant/1 -> Dot Product/1, v_S/1
  Saturation/1 -> Gain/1
  v_Sunb/1 -> Dot Product/2
  Dot Product/1 -> Product/1
  Product/1 -> Saturation/1
  light/1 -> Product/2

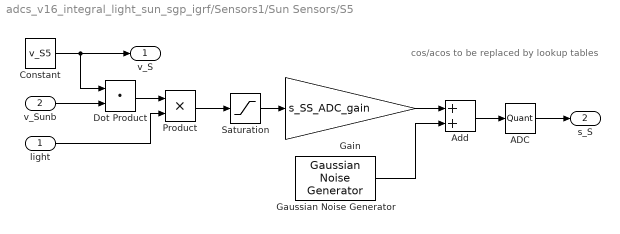
== system adcs_v16_integral_light_sun_sgp_igrf/Sensors1/Sun Sensors/S5 ==
  note: cos/acos to be replaced by lookup tables
  light : Inport  OutDataType=sfix(16)  OutScaling=2^0
  v_Sunb : Inport  Port=2  OutDataType=sfix(16)  OutScaling=2^0
  ADC : Quantizer  QuantizationInterval=1/s_SS_ADC_res
  Add : Sum  OutDataType=sfix(16)  OutScaling=2^-10
  Constant : Constant  Value=v_S5  OutDataType=sfix(16)  OutScaling=2^0
  Dot Product : DotProduct  OutDataType=sfix(16)  OutScaling=2^-10  InputSameDT=on  OutDataTypeStr=Inherit: Inherit via internal rule
  Gain : Gain  Gain=s_SS_ADC_gain  ParameterDataType=sfix(16)  ParameterScaling=2^0  OutDataType=sfix(16)  OutScaling=2^0
  Gaussian Noise Generator : commnoisgen2/Gaussian Noise Generator  SystemSampleTime=-1  m=0  d=s_x_SUNSENSOR  s=41  Ts=s_SIM_STEP_SIZE  frameBased=off  sampPerFrame=1  orient=off  outDataType=double
  Product : Product  OutDataType=fixdt(1, 16)  OutScaling=2^0  RndMeth=Zero
  Saturation : Saturate  UpperLimit=inf  LowerLimit=0  OutDataType=sfix(16)  OutScaling=2^0
  v_S : Outport  OutDataType=sfix(16)  OutScaling=2^0
  s_S : Outport  Port=2  OutDataType=sfix(16)  OutScaling=2^0
  wires:
  light/1 -> Product/2
  Product/1 -> Saturation/1
  Dot Product/1 -> Product/1
  v_Sunb/1 -> Dot Product/2
  Saturation/1 -> Gain/1
  Constant/1 -> v_S/1, Dot Product/1
  Gaussian Noise Generator/1 -> Add/2
  Gain/1 -> Add/1
  Add/1 -> ADC/1
  ADC/1 -> s_S/1

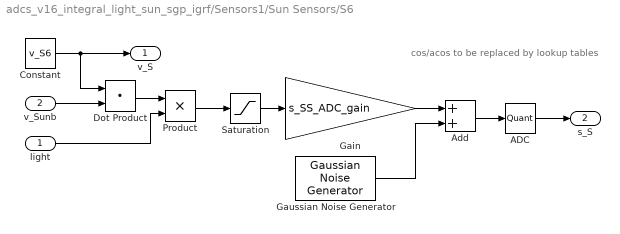
== system adcs_v16_integral_light_sun_sgp_igrf/Sensors1/Sun Sensors/S6 ==
  note: cos/acos to be replaced by lookup tables
  light : Inport  OutDataType=sfix(16)  OutScaling=2^0
  v_Sunb : Inport  Port=2  OutDataType=sfix(16)  OutScaling=2^0
  ADC : Quantizer  QuantizationInterval=1/s_SS_ADC_res
  Add : Sum  OutDataType=sfix(16)  OutScaling=2^-10
  Constant : Constant  Value=v_S6  OutDataType=sfix(16)  OutScaling=2^0
  Dot Product : DotProduct  OutDataType=sfix(16)  OutScaling=2^-10  InputSameDT=on  OutDataTypeStr=Inherit: Inherit via internal rule
  Gain : Gain  Gain=s_SS_ADC_gain  ParameterDataType=sfix(16)  ParameterScaling=2^0  OutDataType=sfix(16)  OutScaling=2^0
  Gaussian Noise Generator : commnoisgen2/Gaussian Noise Generator  SystemSampleTime=-1  m=0  d=s_x_SUNSENSOR  s=41  Ts=s_SIM_STEP_SIZE  frameBased=off  sampPerFrame=1  orient=off  outDataType=double
  Product : Product  OutDataType=fixdt(1, 16)  OutScaling=2^0  RndMeth=Zero
  Saturation : Saturate  UpperLimit=inf  LowerLimit=0  OutDataType=sfix(16)  OutScaling=2^0
  v_S : Outport  OutDataType=sfix(16)  OutScaling=2^0
  s_S : Outport  Port=2  OutDataType=sfix(16)  OutScaling=2^0
  wires:
  ADC/1 -> s_S/1
  Add/1 -> ADC/1
  Gain/1 -> Add/1
  Gaussian Noise Generator/1 -> Add/2
  Constant/1 -> Dot Product/1, v_S/1
  Saturation/1 -> Gain/1
  v_Sunb/1 -> Dot Product/2
  Dot Product/1 -> Product/1
  Product/1 -> Saturation/1
  light/1 -> Product/2

== matlab function Torquer/Embedded MATLAB Function4 ==
  data: euler input double; DCM output double
function DCM  = f(euler)
% This block supports the Embedded MATLAB subset.
% See the help menu for details. 

roll = euler(1);
pitch = euler(2);
yaw = euler(3);

rot_x = [  1         0           0;...
             0         cos(roll)  sin(roll);...
             0        -sin(roll)  cos(roll)];
         
rot_y = [cos(pitch)   0       -sin(pitch);...
            0           1        0;...
           sin(pitch)   0        cos(pitch)];
       
rot_z = [ cos(yaw) sin(yaw) 0;...
           -sin(yaw) cos(yaw) 0;...
            0        0            1];
         
DCM  = rot_z *  rot_y *  rot_x;

== matlab function Embedded MATLAB Function ==
  data: x input double; u input double; xdot output double; m_INERTIA parameter double
function xdot = fcn(x, u, m_INERTIA)
% This block supports the Embedded MATLAB subset.
% See the help menu for details. 

q = x(1:4);
w = x(5:7);

W = ...
    [ 0 w(3) -w(2) w(1);
      -w(3) 0 w(1) w(2);
      w(2) -w(1) 0 w(3);
      -w(1) -w(2) -w(3) 0];
  
  qdot = 0.5 * W * q;
  wdot = inv(m_INERTIA)*( u - cross( w, m_INERTIA*w ) );
  
  xdot = [qdot; wdot];

== matlab function Subsystem/Sun Vector Propagator ==
  data: today input double; v_Sun_i output double; t input double; equinox input double
function v_Sun_i = fcn(today,t,equinox)
% This sun model block gives the sun vector in body frame.
% See the help menu for details. 

% beta = 0;   %what is this? document this block.
% time1 = today + t / 86400;
% lambda = (2*pi*time1) / 365.256363;
% epsilon = 23.5 * pi / 180;
% 
% sin_delta = cos(epsilon)*sin(beta) + sin(epsilon)*cos(beta)*sin(lambda);
% delta = asin(sin_delta);
% 
% cos_alpha = cos(lambda) * cos(beta) / cos(delta);
% alpha = acos(cos_alpha);
% if (delta >= 0)
%     alpha = alpha;
% else
%     alpha = (2*pi - 2*alpha) + alpha;
% end
% 
% x = cos(delta)*cos(alpha);
% y = cos(delta)*sin(alpha);
% z = sin(delta);
% 
% v_Sun_i = [x; y; z];

% taken from sun_calc.m
%     equinox = datenum('21-Mar-2010 12:0:0'); % date of equinox

%//new one
%     beta = 0;   %what is this? document this block.
%     time1 = today - equinox + t / 86400;
%     lambda = (2*pi*time1) / 365.256363;
%     epsilon = 23.5 * pi / 180;
% 
%     sin_delta = cos(epsilon)*sin(beta) + sin(epsilon)*cos(beta)*sin(lambda);
%     delta = asin(sin_delta);
% 
%     cos_alpha = cos(lambda) * cos(beta) / cos(delta);
%     alpha = acos(cos_alpha);
%     if (delta >= 0)
%         alpha = alpha;
%     else
%         alpha = (2*pi - 2*alpha) + alpha;
%     end
% 
%     x = cos(delta)*cos(alpha);
%     y = cos(delta)*sin(alpha);
%     z = sin(delta);
% 
%     v_Sun_i = [x; y; z];

t1 = today - equinox + t / 86400;
l = 2*pi*t1 / 365.256363;
e = 23.45 * pi / 180;

x = cos(l);
y = sin(l)*cos(e);
z = sin(l)*sin(e);

v_Sun_i = [x; y; z];

== matlab function Subsystem/f: I->B ==
  data: x input double; v_B output double; v_I input double
function v_B = fcn(x, v_I)
% This block supports the Embedded MATLAB subset.
% See the help menu for details. 

q = x(1:4);

q0 = q(4); q1 = q(1); q2 = q(2); q3 = q(3);

TBI = [ q0^2 + q1^2 - q2^2 - q3^2,         2*q0*q3 + 2*q1*q2,         2*q1*q3 - 2*q0*q2;
           2*q1*q2 - 2*q0*q3, q0^2 - q1^2 + q2^2 - q3^2,         2*q0*q1 + 2*q2*q3;
           2*q0*q2 + 2*q1*q3,         2*q2*q3 - 2*q0*q1, q0^2 - q1^2 - q2^2 + q3^2];

v_B =  TBI*v_I;
v_B = v_B/sqrt(dot(v_B,v_B));

== matlab function I -> B/L_Inertial ==
  data: x input double; v_B output double; v_I input double
function v_B = fcn(x, v_I)
% This block supports the Embedded MATLAB subset.
% See the help menu for details. 

q = x(1:4);

q0 = q(4); q1 = q(1); q2 = q(2); q3 = q(3);

TBI = [ q0^2 + q1^2 - q2^2 - q3^2,         2*q0*q3 + 2*q1*q2,         2*q1*q3 - 2*q0*q2;
           2*q1*q2 - 2*q0*q3, q0^2 - q1^2 + q2^2 - q3^2,         2*q0*q1 + 2*q2*q3;
           2*q0*q2 + 2*q1*q3,         2*q2*q3 - 2*q0*q1, q0^2 - q1^2 - q2^2 + q3^2];

v_B =  TBI*v_I;

== matlab function q -> w/Subsystem6/(1-L) + L/z ==
  data: a input double; y output double; b input double
function y = fcn(a,b)
%#eml

c = 1-a;

y = c+b;
if y>1
    y=1;
end

== matlab function q-normalise ==
  data: x input double; xN output double
function xN  = fcn(x)
% This block gives DCM for converting from ECI to ORBIT frames
% inputs: state vector in ECI
% output: DCM

q = x(1:4);
q = q/sqrt(dot(q,q));
xN = [q; x(5:7)];
